simulink model "x35BusNetworkElectricityTransmissionModel"  (R2023b)
settings: Solver=VariableStepAuto  StartTime=0.0  StopTime=0.8  RelTol=1e-3
model workspace (MAT data in the model file):
  Compensation_Ki = 30
  Compensation_Kp = 3
  DC_Ki = 400
  DC_Kp = 8
  F = 0.01
  Flux_min = 0.5
  Grid_Freq_PWM = 2700
  Grid_Ireg_Ki = 5
  Grid_Ireg_Kp = 0.83
  Grid_Ireg_lim = 1.1
  Grid_Modindex_Upper = 1.1
  Grid_conv_Imax = 0.8
  H = 0.685
  Idref_max = 0.9
  Iqref_Tc = 0.3
  Ki_Var = 0.05
  Ki_Vreg = 20
  Ksh = 1.1
  L_pu = 0.3
  Llr = 0.16
  Lls = 0.18
  Lm = 2.9
  Nb_wt = 6
  P_mech = 1080000
  Pitch_Ki = 0
  Pitch_Kp = 150
  Pitch_Max = 27
  Pitch_Tc = 0.01
  Pitch_rate = 10
  Q_Filt = 50
  R_pu = 0.003
  Rotor_Freq_PWM = 1620
  Rotor_Ireg_Ki = 8
  Rotor_Ireg_Kp = 0.6
  Rotor_Ireg_lim = 0.1
  Rotor_Modindex_Upper = 2
  Rr = 0.016
  Rs = 0.023
  T_set = 0.0001
  Tp = 5e-05
  Ts = 5e-06
  Var_C_Filt = 720000
  Var_reg_max = 1.1
  Var_reg_min = 0.9
  WT_Coeff = [0.645 116 0.4 5 21 0.00912 0.08 0.035]
  WT_H = 4.32
  WT_IGBTRon = 5.931
  WT_Param = [91.204 10143]
  Wind_Freq_Filt = 10000
  Wind_Freq_nom = 60
  Wind_P_nom = 1200000
  Wind_Rotor_V_nom = 1950
  Wind_V_nom = 500
  Zeta_Filt = 0.707106781187
  init = [-0.2 0 0 0 0 0 0 0]
  p = 3
  torque0 = 0.83
  v_Ki = 0.1
  v_Kp = 3.6
  v_Max = 1.2
  v_Min = 0.7
  v_T = 5
  vreg_max = 1
  wind_VDC_nom = 1150
  wt0 = 1.2
undefined symbols (not defined in the file): D1, D11, Delta, DiscIntNeverNeededParam, Ion, Lithium, P, Q
libraries: powerlib_extras x144, spsSeriesRLCBranchLib x67, spsLoadFlowBusLib x43, spsThreePhaseTransformerTwoWindingsLib x32, spsThreePhaseSeriesRLCLoadLib x31, spsThreePhaseVIMeasurementLib x26, simulink_extras x26, spsDistributedParametersLineLib x22, spsGenericPowerSystemStabilizerLib x20, spsSynchronousMachinepuStandardLib x10, spsExcitationSystemLib x10, spsHydraulicTurbineandGovernorLib x10
(part 3 of 16)

== system x35BusNetworkElectricityTransmissionModel/North Network ==
  1320 MVar : spsThreePhaseSeriesRLCLoadLib/Three-Phase Series RLC Load  LConnTagsString=A|B|C  Configuration=Y (grounded)  NominalVoltage=650e3  Vabc=[1e3 1e3 1e3]  Vabcp=[1e3 1e3 1e3]  NominalFrequency=60  UnbalancedPower=off  ActivePower=4400e3  InductivePower=1320e6  CapacitivePower=0  Pabc=[10e3 9e3 11e3]  QLabc=[100 90 110]  QCabc=[100 90 110]  Pabcp=[10e3 9e3 11e3]  QLabcp=[100 90 110]  QCabcp=[100 90 110]  Measurements=None  LoadType=constant Z
  135 MW : spsThreePhaseSeriesRLCLoadLib/Three-Phase Series RLC Load  LConnTagsString=A|B|C  Configuration=Y (grounded)  NominalVoltage=17e3  Vabc=[1e3 1e3 1e3]  Vabcp=[1e3 1e3 1e3]  NominalFrequency=60  UnbalancedPower=off  ActivePower=135e6  InductivePower=0  CapacitivePower=0  Pabc=[10e3 9e3 11e3]  QLabc=[100 90 110]  QCabc=[100 90 110]  Pabcp=[10e3 9e3 11e3]  QLabcp=[100 90 110]  QCabcp=[100 90 110]  Measurements=None  LoadType=constant Z
  155 MW : spsThreePhaseSeriesRLCLoadLib/Three-Phase Series RLC Load  LConnTagsString=A|B|C  Configuration=Y (grounded)  NominalVoltage=17e3  Vabc=[1e3 1e3 1e3]  Vabcp=[1e3 1e3 1e3]  NominalFrequency=60  UnbalancedPower=off  ActivePower=155e6  InductivePower=0  CapacitivePower=0  Pabc=[10e3 9e3 11e3]  QLabc=[100 90 110]  QCabc=[100 90 110]  Pabcp=[10e3 9e3 11e3]  QLabcp=[100 90 110]  QCabcp=[100 90 110]  Measurements=None  LoadType=constant Z
  1980 MVar : spsThreePhaseSeriesRLCLoadLib/Three-Phase Series RLC Load  LConnTagsString=A|B|C  Configuration=Y (grounded)  NominalVoltage=650e3  Vabc=[1e3 1e3 1e3]  Vabcp=[1e3 1e3 1e3]  NominalFrequency=60  UnbalancedPower=off  ActivePower=6600e3  InductivePower=1980e6  CapacitivePower=0  Pabc=[10e3 9e3 11e3]  QLabc=[100 90 110]  QCabc=[100 90 110]  Pabcp=[10e3 9e3 11e3]  QLabcp=[100 90 110]  QCabcp=[100 90 110]  Measurements=None  LoadType=constant Z
  205 MW : spsThreePhaseSeriesRLCLoadLib/Three-Phase Series RLC Load  LConnTagsString=A|B|C  Configuration=Y (grounded)  NominalVoltage=17e3  Vabc=[1e3 1e3 1e3]  Vabcp=[1e3 1e3 1e3]  NominalFrequency=60  UnbalancedPower=off  ActivePower=205e6  InductivePower=0  CapacitivePower=0  Pabc=[10e3 9e3 11e3]  QLabc=[100 90 110]  QCabc=[100 90 110]  Pabcp=[10e3 9e3 11e3]  QLabcp=[100 90 110]  QCabcp=[100 90 110]  Measurements=None  LoadType=constant Z
  "2700 MVA 17KV :650KV Transformer " : spsThreePhaseTransformerTwoWindingsLib/Three-Phase Transformer (Two Windings)  Winding1Connection=Yg  Winding2Connection=Delta (D1)  CoreType=Three single-phase transformers  SetSaturation=off  Hysteresis=off  DataFile='hysteresis'  SetInitialFlux=off  Measurements=None  UNITS=pu  NominalPower=[ 2700e6 , 60 ]  Winding1=[650e3 , 0.002 , 0.08 ]  Winding2=[17e3 , 0.002 , 0.08 ]  Rm=500  Lm=500  L0=0.5  Saturation=[ 0,0 ; 0.0024,1.2 ; 1.0,1.52 ]  InitialFluxes=[ 0.8 , -0.8 , 0.7 ]  BreakLoop=off  DiscreteSolver=Trapezoidal iterative  DataType=off  TransfoNumber=1
  "3100 MVA 17KV :650KV Transformer " : spsThreePhaseTransformerTwoWindingsLib/Three-Phase Transformer (Two Windings)  Winding1Connection=Yg  Winding2Connection=Delta (D1)  CoreType=Three single-phase transformers  SetSaturation=off  Hysteresis=off  DataFile='hysteresis'  SetInitialFlux=off  Measurements=None  UNITS=pu  NominalPower=[ 3100e6 , 60 ]  Winding1=[ 650e3 , 0.002 , 0.08 ]  Winding2=[ 17e3 , 0.002 , 0.08 ]  Rm=500  Lm=500  L0=0.5  Saturation=[ 0,0 ; 0.0024,1.2 ; 1.0,1.52 ]  InitialFluxes=[ 0.8 , -0.8 , 0.7 ]  BreakLoop=off  DiscreteSolver=Trapezoidal iterative  DataType=off  TransfoNumber=1
  "4100 MVA 17KV :650KV Transformer " : spsThreePhaseTransformerTwoWindingsLib/Three-Phase Transformer (Two Windings)  Winding1Connection=Yg  Winding2Connection=Delta (D1)  CoreType=Three single-phase transformers  SetSaturation=off  Hysteresis=off  DataFile='hysteresis'  SetInitialFlux=off  Measurements=None  UNITS=pu  NominalPower=[ 4100e6 , 60 ]  Winding1=[ 650e3 , 0.002 , 0.08 ]  Winding2=[ 17e3 , 0.002 , 0.08 ]  Rm=500  Lm=500  L0=0.5  Saturation=[ 0,0 ; 0.0024,1.2 ; 1.0,1.52 ]  InitialFluxes=[ 0.8 , -0.8 , 0.7 ]  BreakLoop=off  DiscreteSolver=Trapezoidal iterative  DataType=off  TransfoNumber=1
  660 MVar : spsThreePhaseSeriesRLCLoadLib/Three-Phase Series RLC Load  LConnTagsString=A|B|C  Configuration=Y (grounded)  NominalVoltage=650e3  Vabc=[1e3 1e3 1e3]  Vabcp=[1e3 1e3 1e3]  NominalFrequency=60  UnbalancedPower=off  ActivePower=2200e3  InductivePower=660e6  CapacitivePower=0  Pabc=[10e3 9e3 11e3]  QLabc=[100 90 110]  QCabc=[100 90 110]  Pabcp=[10e3 9e3 11e3]  QLabcp=[100 90 110]  QCabcp=[100 90 110]  Measurements=None  LoadType=constant Z
  990 Mvar : spsThreePhaseParallelRLCLoadLib/Three-Phase Parallel RLC Load  LConnTagsString=A|B|C  Configuration=Y (grounded)  NominalVoltage=650e3  Vabc=[1e3 1e3 1e3]  Vabcp=[1e3 1e3 1e3]  NominalFrequency=60  UnbalancedPower=off  ActivePower=3300e3  InductivePower=990e6  CapacitivePower=0  Pabc=[10e3 9e3 11e3]  QLabc=[100 90 110]  QCabc=[100 90 110]  Pabcp=[10e3 9e3 11e3]  QLabcp=[100 90 110]  QCabcp=[100 90 110]  Measurements=None  LoadType=constant Z
  ATL-CAD 447 km : spsDistributedParametersLineLib/Distributed Parameters Line  Phases=3  Length=447  Frequency=60  Resistance=[0.01273 0.3864]/6  Inductance="[0.9337e-3  4.1264e-3]/6"  Capacitance=[12.74e-9 7.751e-9]*6  x1=[-0.00258 1.64377320763255e-08 -194904.094021767 -120223.665929989;-0.00252 1.80656414411054e-08 -192135.055279541 -124601.181939555;-0.00246 1.96843080899094e-08 -189267.716692787 -128914.949682076;-0.0024 2.12929038829704e-08 -186303.545244907 -133162.762154265;-0.00234 2.28906058329572e-08 -183244.057460786 -137342.44609677;-0.00228 2.44765965260301e-08 -180090.818630907 -141451.863106056;-0.00222 2.60500645400448e-08 -176845.442010521 -145488.910728447;-0.00216 2.7610204859691e-08 -173509.587994275 -149451.523535784;-0.0021 2.9156219288353e-08 -170084.963266721 -153337.674182133;-0.00204 3.06873168564822e-08 -166573.319929152 -157145.374441016;-0.00198 3.22027142262711e-08 -162976.454603186 -160872.676222622;-0.00192 3.37016360924241e-08 -159296.207511587 -164517.672570487;-0.00186 3.51833155788176e-08 -155534.461536769 -168078.498637129;-0.0018 3.6646994630848e-08 -151693.141257482 -171553.332638133;-0.00174 3.80919244032667e-08 -147774.211964161 -174940.39678422;-0.00168 3.95173656433029e-08 -143779.678653446 -178237.958190784;-0.00162 4.09225890688789e-08 -139711.585002389 -181444.329764479;-0.00156 4.23068757417249e-08 -135572.012322871 -184557.871066362;-0.0015 4.36695174352002e-08 -131363.078496766 -187576.989151169;-0.00144 4.50098169966357e-08 -127086.936892391 -190500.139382302;-0.00138 4.632708870401e-08 -122745.775262806 -193325.826222089;-0.00132 4.76206586167771e-08 -118341.814626515 -196052.603996931;-0.00126 4.88898649206673e-08 -113877.308131156 -198679.077636932;-0.0012 5.01340582662832e-08 -109354.539900746 -201203.903389647;-0.00114 5.13526021013192e-08 -104775.823867084 -203625.789507567;-0.00108 5.25448729962332e-08 -100143.502585896 -205943.496909003;-0.00102 5.37102609632047e-08 -95459.9460383467 -208155.839812022;-0.00096 5.48481697682159e-08 -90727.5504185068 -210261.686341115;-0.0009 5.5958017236096e-08 -85948.7369074205 -212259.959106288;-0.00084 5.70392355483729e-08 -81125.9504343822 -214149.635754268;-0.00078 5.80912715337793e-08 -76261.6584260665 -215929.749491566;-0.00072 5.91135869512658e-08 -71358.3495441466 -217599.389579101;-0.00066 6.01056587653745e-08 -66418.5324120493 -219157.701798153;-0.0006 6.1066979413834e-08 -61444.7343314965 -220603.888887397;-0.00054 6.19970570672373e-08 -56439.4999894916 -221937.210950794;-0.00048 6.28954158806711e-08 -51405.39015641 -223156.985836141;-0.00042 6.37615962371667e-08 -46344.980375862 -224262.589484067;-0.00036 6.45951549828486e-08 -41260.859646997 -225253.456247317;-0.0003 6.53956656536599e-08 -36155.6290999235 -226129.079180146;-0.00024 6.61627186935499e-08 -31031.9006649233 -226889.010297681;-0.00018 6.68959216640098e-08 -25892.2957361393 -227532.86080512;-0.00012 6.75948994448519e-08 -20739.4438304221 -228060.301296648;-6e-05 6.82592944261279e-08 -15575.9812420204 -228471.061923963]  x2=[-0.00258 4.87559476940855e-09 -301606.612191046 -117006.023986347;-0.00252 5.95262307883651e-09 -298883.042776193 -123797.71586053;-0.00246 7.02660591630551e-09 -296006.559273932 -130526.070535761;-0.0024 8.09699381235099e-09 -292978.633346374 -137187.64566146;-0.00234 9.16323913674683e-09 -289800.814136373 -143779.033052703;-0.00228 1.02247963786831e-08 -286474.727474956 -150296.860433905;-0.00222 1.12811224258595e-08 -283002.07504952 -156737.793164143;-0.00216 1.23316768423517e-08 -279384.63353321 -163098.535943216;-0.0021 1.33759221451082e-08 -275624.253675951 -169375.834497586;-0.00204 1.44133240789366e-08 -271722.85935756 -175566.477245322;-0.00198 1.54433518898386e-08 -267682.446603461 -181667.296939203;-0.00192 1.64654785965534e-08 -263505.082563477 -187675.172287145;-0.00186 1.74791812601711e-08 -259192.904454239 -193587.029549106;-0.0018 1.84839412516781e-08 -254748.118465748 -199399.844109673;-0.00174 1.94792445172967e-08 -250172.998632646 -205110.642025508;-0.00168 2.04645818414852e-08 -245469.885670778 -210716.501546873;-0.00162 2.14394491074616e-08 -240641.185779639 -216214.554612454;-0.00156 2.24033475551191e-08 -235689.369411317 -221601.98831671;-0.0015 2.33557840362012e-08 -230616.970006566 -226876.046349009;-0.00144 2.42962712666051e-08 -225426.582698647 -232034.030403808;-0.00138 2.52243280756855e-08 -220120.862985616 -237073.301561157;-0.00132 2.61394796524304e-08 -214702.525371715 -241991.281636816;-0.00126 2.70412577883831e-08 -209174.341978588 -246785.454501306;-0.0012 2.79292011171863e-08 -203539.141127007 -251453.367367201;-0.00114 2.88028553506256e-08 -197799.805889854 -255992.632044027;-0.00108 2.96617735110519e-08 -191959.272617088 -260400.9261601;-0.00102 3.05055161600635e-08 -186020.529433451 -264675.994350693;-0.00096 3.13336516233304e-08 -179986.614709693 -268815.649411926;-0.0009 3.21457562114475e-08 -173860.615508078 -272817.773419778;-0.00084 3.29414144367015e-08 -167645.666002995 -276680.318813656;-0.00078 3.37202192256424e-08 -161344.945877449 -280401.309443964;-0.00072 3.44817721273494e-08 -154961.67869628 -283978.84158314;-0.00066 3.52256835172862e-08 -148499.130256927 -287411.084899637;-0.0006 3.59515727966398e-08 -141960.606918587 -290696.283394352;-0.00054 3.66590685870419e-08 -135349.453910617 -293832.756299034;-0.00048 3.73478089205732e-08 -128669.053621055 -296818.898936187;-0.00042 3.80174414249525e-08 -121922.823866131 -299653.183540063;-0.00036 3.86676235038173e-08 -115114.216141641 -302334.160038285;-0.0003 3.9298022512002e-08 -108246.713857108 -304860.456793738;-0.00024 3.99083159257256e-08 -101323.830553596 -307230.781306322;-0.00018 4.04981915076007e-08 -94349.1081061232 -309443.920874218;-0.00012 4.106734746638e-08 -87326.1149115726 -311498.743214328;-6e-05 4.16154926113581e-08 -80258.4440630321 -313394.197041575]  x3=[-0.00258 2.91635300112185e-11 -5053.27339398635 2918.21649596622;-0.00252 3.84630024253407e-11 -5117.98290026042 2803.17747700594;-0.00246 4.77427964567074e-11 -5180.07395191326 2686.70430065166;-0.0024 5.69981643912216e-11 -5239.51478201554 2568.85655673258;-0.00234 6.62243710116282e-11 -5296.27497954025 2449.69453833206;-0.00228 7.54166960201396e-11 -5350.3255049215 2329.27921094058;-0.00222 8.45704364534267e-11 -5401.6387049118 2207.67218126465;-0.00216 9.36809090887422e-11 -5450.18832672985 2084.9356657077;-0.0021 1.02743452839944e-10 -5495.94953149205 1961.13245853899;-0.00204 1.11753431142192e-10 -5538.89890692046 1836.32589976693;-0.00198 1.20706234324102e-10 -5579.01447932101 1710.57984273314;-0.00192 1.29597281966136e-10 -5616.2757248256 1583.95862144394;-0.00186 1.38422025244034e-10 -5650.66357989254 1456.52701765581;-0.0018 1.47175949256073e-10 -5682.16045105973 1328.35022773192;-0.00174 1.55854575332973e-10 -5710.75022394592 1199.49382928644;-0.00168 1.64453463329272e-10 -5736.418271495 1070.0237476338;-0.00162 1.7296821389498e-10 -5759.15146145956 940.006222060097;-0.00156 1.81394470726375e-10 -5778.93816311956 809.507771933874;-0.0015 1.89727922794762e-10 -5795.7682532328 678.595162673546;-0.00144 1.97964306552078e-10 -5809.63312121421 547.335371588997;-0.00138 2.06099408112202e-10 -5820.52567354113 415.795553614749;-0.00132 2.14129065406857e-10 -5828.44033738251 284.043006952253;-0.00126 2.22049170315e-10 -5833.37306345009 152.145138638889;-0.0012 2.29855670764612e-10 -5835.32132807008 20.1694300612777;-0.00114 2.37544572805817e-10 -5834.28413447428 -111.816597569441;-0.00108 2.45111942654255e-10 -5830.26201331011 -243.745417762709;-0.00102 2.52553908703683e-10 -5823.25702236907 -375.549533296353;-0.00096 2.59866663506759e-10 -5813.27274553397 -507.161510749404;-0.0009 2.67046465723001e-10 -5800.31429094533 -638.51401500229;-0.00084 2.74089642032928e-10 -5784.38828838795 -769.539843686717;-0.00078 2.80992589017397e-10 -5765.50288589903 -900.171961567653;-0.00072 2.87751775001178e-10 -5743.66774559943 -1030.34353483979;-0.00066 2.94363741859827e-10 -5718.89403875042 -1159.98796532093;-0.0006 3.00825106788924e-10 -5691.19444003816 -1289.03892452491;-0.00054 3.07132564034779e-10 -5660.5831210892 -1417.4303875964;-0.00048 3.13282886585716e-10 -5627.07574321994 -1545.0966670905;-0.00042 3.19272927823074e-10 -5590.68944942404 -1671.9724465796;-0.00036 3.25099623131072e-10 -5551.44285560176 -1797.99281407054;-0.0003 3.30759991464727e-10 -5509.35604103568 -1923.09329521471;-0.00024 3.36251136875005e-10 -5464.45053811781 -2047.20988629437;-0.00018 3.41570249990452e-10 -5416.7493213332 -2170.27908696812;-0.00012 3.46714609454512e-10 -5366.27679550578 -2292.23793275882;-6e-05 3.51681583317825e-10 -5313.05878331239 -2413.02402726744]  x4=[-0.00258 -3.35866188879571e-10 -7329.89893613951 -4834.75933302617;-0.00252 -3.24943372678954e-10 -7218.67296251981 -4999.30757604478;-0.00246 -3.13854309444611e-10 -7103.75378242676 -5161.29808093091;-0.0024 -3.02604672546196e-10 -6985.20019063633 -5320.647970349;-0.00234 -2.91200217505814e-10 -6863.07284135671 -5477.2757179512;-0.00228 -2.79646779053395e-10 -6737.43421719646 -5631.10119008767;-0.00222 -2.67950268141535e-10 -6608.34859719721 -5782.04568680451;-0.00216 -2.56116668921341e-10 -6475.8820239474 -5930.03198210806;-0.0021 -2.44152035680835e-10 -6340.10226979359 -6074.98436347517;-0.00204 -2.32062489747464e-10 -6201.07880216694 -6216.82867058912;-0.00198 -2.19854216356316e-10 -6058.88274804233 -6355.49233328141;-0.00192 -2.07533461485642e-10 -5913.58685754855 -6490.90440866;-0.00186 -1.95106528661294e-10 -5765.26546674792 -6622.99561740499;-0.0018 -1.82579775731729e-10 -5613.99445960465 -6751.69837921324;-0.00174 -1.69959611615213e-10 -5459.85122916116 -6876.94684737363;-0.00168 -1.57252493020902e-10 -5302.91463794237 -6998.67694245554;-0.00162 -1.4446492114547e-10 -5143.26497760822 -7116.82638509301;-0.00156 -1.31603438346975e-10 -4980.98392787491 -7231.33472784804;-0.0015 -1.1867462479767e-10 -4816.1545147261 -7342.14338613659;-0.00144 -1.05685095117463e-10 -4648.86106793525 -7449.19566820159;-0.00138 -9.26414949897582e-11 -4479.18917792097 -7552.43680411743;-0.00132 -7.95504977613986e-11 -4307.22565195737 -7651.81397381129;-0.00126 -6.641880102846e-11 -4133.05846976185 -7747.27633408688;-0.0012 -5.3253123209637e-11 -3956.77673848305 -7838.77504463675;-0.00114 -4.00602001089753e-11 -3778.47064711202 -7926.26329302987;-0.00108 -2.68467814697105e-11 -3598.23142033982 -8009.69631866178;-0.00102 -1.36196275209744e-11 -3416.1512718853 -8089.03143565488;-0.00096 -3.85505519136652e-13 -3232.32335731687 -8164.22805469739;-0.0009 1.2848813714448e-11 -3046.84172639237 -8235.24770380952;-0.00084 2.60765592575175e-11 -2859.80127494148 -8302.05404802651;-0.00078 3.92909635510314e-11 -2671.29769631527 -8364.6129079882;-0.00072 5.24852658615791e-11 -2481.42743242773 -8422.89227742589;-0.00066 6.56527157402959e-11 -2290.28762441425 -8476.8623395373;-0.0006 7.87865764765172e-11 -2097.97606293247 -8526.49548224139;-0.00054 9.18801285444045e-11 -1904.59113813076 -8571.76631230524;-0.00048 1.04926673040779e-10 -1710.23178930997 -8612.65166833569;-0.00042 1.17919535112404e-10 -1514.99745430433 -8649.13063262912;-0.00036 1.30852067370963e-10 -1318.98801860713 -8681.18454187333;-0.0003 1.43717653293986e-10 -1122.30376426752 -8708.79699669608;-0.00024 1.56509710609988e-10 -925.045318584315 -8731.95387005524;-0.00018 1.69221694666074e-10 -727.313602623252 -8750.64331446653;-0.00012 1.81847101776312e-10 -529.209779583876 -8764.85576806484;-6e-05 1.94379472549133e-10 -330.835203042593 -8774.5839594963]  x5=0.00252797080447097  V1=[6.404e-19 2.341e-08 2.341e-08;377 377 377;-1.588 0.8733 -0.6975]  V2=[3.447e-16 8.016e-05 8.016e-05;377 377 377;2.581 0.8892 -0.6816]  I1=[4.995e-19 5.332e-07 5.332e-07;377 377 377;1.203 -0.6479 -2.219]  I2=[4.022e-19 5.225e-07 5.225e-07;377 377 377;-2.95 1.909 0.3385]  nHarmo=1  Measurements=None  Decoupling=off  VsMag0=0  VrMag0=0  VsAngle0=0  VrAngle0=0  IsMag0=0  IrMag0=0  IsAngle0=0  IrAngle0=0
      settings: LibrarySourceBlock=sps_lib/Power Grid Elements/Distributed Parameters Line
  BMW 1 : spsThreePhaseVIMeasurementLib/Three-Phase V-I Measurement  VoltageMeasurement=no  SetLabelV=off  LabelV=Vabc  Vpu=off  VpuLL=off  CurrentMeasurement=no  SetLabelI=off  LabelI=Iabc  Ipu=off  Pbase=100e6  Vbase=500e3  OutputType=Complex  PhasorSimulation=off  PSBequivalent=0
  BMW- FER 131 km : spsDistributedParametersLineLib/Distributed Parameters Line  Phases=3  Length=131  Frequency=60  Resistance=[0.01273 0.3864]/6  Inductance="[0.9337e-3  4.1264e-3]/6"  Capacitance=[12.74e-9 7.751e-9]*6  x1=[-0.00078 5.80912715337793e-08 -76261.6584260665 -215929.749491566;-0.00072 5.91135869512658e-08 -71358.3495441466 -217599.389579101;-0.00066 6.01056587653745e-08 -66418.5324120492 -219157.701798153;-0.0006 6.1066979413834e-08 -61444.7343314965 -220603.888887397;-0.00054 6.19970570672373e-08 -56439.4999894916 -221937.210950794;-0.00048 6.28954158806711e-08 -51405.39015641 -223156.985836141;-0.00042 6.37615962371667e-08 -46344.980375862 -224262.589484067;-0.00036 6.45951549828486e-08 -41260.859646997 -225253.456247317;-0.0003 6.53956656536599e-08 -36155.6290999235 -226129.079180146;-0.00024 6.61627186935499e-08 -31031.9006649233 -226889.010297681;-0.00018 6.68959216640098e-08 -25892.2957361393 -227532.86080512;-0.00012 6.75948994448519e-08 -20739.4438304221 -228060.301296648;-6e-05 6.82592944261279e-08 -15575.9812420204 -228471.061923963]  x2=[-0.00078 2.91154256756996e-08 -40332.3471165906 -195014.245406608;-0.00072 3.00931854241187e-08 -35911.2883875951 -195876.599881198;-0.00066 3.10555489428166e-08 -31471.8567798962 -196638.740267906;-0.0006 3.20020238688349e-08 -27016.3235887357 -197300.276641627;-0.00054 3.29321259681124e-08 -22546.9683472229 -197860.870548128;-0.00048 3.3845379383229e-08 -18066.0776600836 -198320.235177208;-0.00042 3.47413168768623e-08 -13575.9440337906 -198678.135509435;-0.00036 3.56194800708358e-08 -9078.86470367538 -198934.388436385;-0.0003 3.64794196806327e-08 -4577.1404586196 -199088.862854326;-0.00024 3.73206957452588e-08 -73.0744639293679 -199141.479731292;-0.00018 3.81428778523344e-08 4431.02891700687 -199092.212147516;-0.00012 3.89455453583015e-08 8932.86530167318 -198941.085309204;-6e-05 3.97282876036323e-08 13430.1314673908 -198688.17653564]  x3=[-0.00078 2.7051916331608e-10 801.205877154994 -9199.13249771914;-0.00072 2.61865618398496e-10 1009.06227174107 -9178.65876986299;-0.00066 2.53078098191819e-10 1216.40241142359 -9153.48907057806;-0.0006 2.44161098553761e-10 1423.1202171559 -9123.63627714759;-0.00054 2.35119181586105e-10 1629.10992828887 -9089.11566281232;-0.00048 2.25956973300646e-10 1834.26615668004 -9049.9448889564;-0.00042 2.16679161252442e-10 2038.48394061211 -9006.14399607155;-0.00036 2.07290492141571e-10 2241.65879849331 -8957.73539350389;-0.0003 1.97795769384632e-10 2443.68678231211 -8904.743847989;-0.00024 1.8819985065723e-10 2644.46453081894 -8847.19647098073;-0.00018 1.78507645408699e-10 2843.88932240772 -8785.12270478051;-0.00012 1.68724112350334e-10 3041.85912767011 -8718.55430747412;-6e-05 1.58854256918428e-10 3238.2726615957 -8647.52533668367]  x4=[-0.00078 3.05744357291441e-10 -4148.52157769771 353.308180522301;-0.00072 3.32262569637252e-10 -4155.45083096756 259.388186850742;-0.00066 3.5861079031293e-10 -4160.25407880839 165.335485389847;-0.0006 3.84775539081918e-10 -4162.92886378985 71.1981952395781;-0.00054 4.10743429575277e-10 -4163.4738174425 -22.9755212229666;-0.00048 4.365011761404e-10 -4161.888660958 -117.137482984315;-0.00042 4.62035600638195e-10 -4158.1742053317 -211.239515044916;-0.00036 4.87333639185267e-10 -4152.33235094772 -305.233473066364;-0.0003 5.12382348837641e-10 -4144.36608660672 -399.071268002924;-0.00024 5.37168914212613e-10 -4134.27948799673 -492.704890704785;-0.00018 5.61680654045334e-10 -4122.07771560798 -586.086436480422;-0.00012 5.8590502767678e-10 -4107.76701209269 -679.168129605523;-6e-05 6.09829641469786e-10 -4091.3546990712 -771.902347765934]  x5=0.000740859452764423  V1=[1.271e-18 2.341e-08 2.341e-08;377 377 377;2.226 1.284 -0.2866]  V2=[3.351e-20 3.07e-09 3.07e-09;377 377 377;-0.6702 -1.817 2.896]  I1=[5.66e-21 5.705e-10 5.705e-10;377 377 377;-2.518 2.745 1.174]  I2=[6.071e-21 5.74e-10 5.74e-10;377 377 377;0.8934 -0.2657 -1.836]  nHarmo=1  Measurements=None  Decoupling=off  VsMag0=0  VrMag0=0  VsAngle0=0  VrAngle0=0  IsMag0=0  IrMag0=0  IsAngle0=0  IrAngle0=0
      settings: LibrarySourceBlock=sps_lib/Power Grid Elements/Distributed Parameters Line
  BMW- ORE 215 km : spsDistributedParametersLineLib/Distributed Parameters Line  Phases=3  Length=215  Frequency=60  Resistance=[0.01273 0.3864]/6  Inductance="[0.9337e-3  4.1264e-3]/6"  Capacitance=[12.74e-9 7.751e-9]*6  x1=[-0.00126 4.88898649206673e-08 -113877.308131156 -198679.077636932;-0.0012 5.01340582662832e-08 -109354.539900746 -201203.903389647;-0.00114 5.13526021013192e-08 -104775.823867084 -203625.789507567;-0.00108 5.25448729962332e-08 -100143.502585896 -205943.496909003;-0.00102 5.37102609632047e-08 -95459.9460383467 -208155.839812022;-0.00096 5.48481697682159e-08 -90727.5504185068 -210261.686341115;-0.0009 5.5958017236096e-08 -85948.7369074205 -212259.959106288;-0.00084 5.70392355483729e-08 -81125.9504343822 -214149.635754268;-0.00078 5.80912715337793e-08 -76261.6584260665 -215929.749491566;-0.00072 5.91135869512658e-08 -71358.3495441466 -217599.389579101;-0.00066 6.01056587653745e-08 -66418.5324120492 -219157.701798153;-0.0006 6.1066979413834e-08 -61444.7343314965 -220603.888887397;-0.00054 6.19970570672373e-08 -56439.4999894916 -221937.210950794;-0.00048 6.28954158806711e-08 -51405.39015641 -223156.985836141;-0.00042 6.37615962371667e-08 -46344.980375862 -224262.589484067;-0.00036 6.45951549828486e-08 -41260.859646997 -225253.456247317;-0.0003 6.53956656536599e-08 -36155.6290999235 -226129.079180146;-0.00024 6.61627186935499e-08 -31031.9006649233 -226889.010297681;-0.00018 6.68959216640098e-08 -25892.2957361393 -227532.86080512;-0.00012 6.75948994448519e-08 -20739.4438304221 -228060.301296648;-6e-05 6.82592944261279e-08 -15575.9812420204 -228471.061923963]  x2=[-0.00126 1.36103658168936e-08 -202813.109882575 -207023.441617023;-0.0012 1.38562428628494e-08 -198078.85681003 -211557.646069082;-0.00114 1.40950307989227e-08 -193243.262934264 -215983.613720276;-0.00108 1.4326607456793e-08 -188308.802234456 -220299.080163773;-0.00102 1.45508543575631e-08 -183277.999271879 -224501.837527199;-0.00096 1.4767656772375e-08 -178153.427898286 -228589.735602229;-0.0009 1.49769037811073e-08 -172937.709939083 -232560.682944673;-0.00084 1.51784883291238e-08 -167633.513851954 -236412.647944494;-0.00078 1.53723072820449e-08 -162243.553361628 -240143.659865224;-0.00072 1.55582614785129e-08 -156770.586071485 -243751.809852222;-0.00066 1.57362557809248e-08 -151217.412052721 -247235.251909284;-0.0006 1.59061991241067e-08 -145586.872411774 -250592.203843087;-0.00054 1.6068004561904e-08 -139881.847836765 -253820.948174992;-0.00048 1.62215893116647e-08 -134105.257123683 -256919.833019739;-0.00042 1.63668747965932e-08 -128260.055683077 -259887.272930581;-0.00036 1.65037866859506e-08 -122349.23402801 -262721.749710426;-0.0003 1.66322549330845e-08 -116375.81624406 -265421.81318858;-0.00024 1.6752213811266e-08 -110342.858442142 -267986.081962676;-0.00018 1.68636019473163e-08 -104253.447194943 -270413.244105426;-0.00012 1.69663623530068e-08 -98110.6979577777 -272702.057835829;-6e-05 1.70604424542152e-08 -91917.7534746594 -274851.352154489]  x3=[-0.00126 8.69836358039925e-10 -4039.64980114856 3058.27670176948;-0.0012 8.63889633892926e-10 -4107.7865446866 2966.12730134233;-0.00114 8.57500927846383e-10 -4173.82166872521 2872.46037538009;-0.00108 8.50673508480359e-10 -4237.72138847475 2777.32384561284;-0.00102 8.43410868828756e-10 -4299.45301165785 2680.76638564712;-0.00096 8.3571672459222e-10 -4358.98495523544 2582.83739606364;-0.0009 8.27595012237113e-10 -4416.28676156514 2483.58697914299;-0.00084 8.19049886981548e-10 -4471.32911398403 2383.0659132324;-0.00078 8.10085720669502e-10 -4524.08385180755 2281.3256267666;-0.00072 8.00707099534097e-10 -4574.52398473702 2178.4181719561;-0.00066 7.90918821851205e-10 -4622.62370666841 2074.39619815628;-0.0006 7.80725895484555e-10 -4668.35840889521 1969.31292493106;-0.00054 7.70133535323619e-10 -4711.70469269867 1863.22211482472;-0.00048 7.59147160615579e-10 -4752.64038131906 1756.17804585605;-0.00042 7.47772392192742e-10 -4791.14453130166 1648.23548374868;-0.00036 7.36015049596814e-10 -4827.19744321188 1539.44965391193;-0.0003 7.23881148101518e-10 -4860.7806717138 1429.87621318649;-0.00024 7.11376895635068e-10 -4891.87703500717 1319.5712213693;-0.00018 6.98508689604076e-10 -4920.47062361794 1208.59111253239;-0.00012 6.85283113620527e-10 -4946.54680853782 1096.99266615011;-6e-05 6.71706934133474e-10 -4970.09224870877 984.832978049736]  x4=[-0.00126 -5.19223589158569e-10 -4184.55199868995 -10999.0722268337;-0.0012 -4.99570046723291e-10 -3934.70964350595 -11090.9038546552;-0.00114 -4.79660915021117e-10 -3682.85421816326 -11177.0611711283;-0.00108 -4.59506379931703e-10 -3429.11457655123 -11257.5000965779;-0.00102 -4.39116752887615e-10 -3173.62053655909 -11332.1794769634;-0.00096 -4.18502465598804e-10 -2916.50281365868 -11401.0611049339;-0.0009 -3.97674064715557e-10 -2657.89295402802 -11464.1097393757;-0.00084 -3.7664220643263e-10 -2397.92326724987 -11521.2931234424;-0.00078 -3.55417651037343e-10 -2136.72675861967 -11572.5820010582;-0.00072 -3.34011257404423e-10 -1874.43706109759 -11617.9501318855;-0.00066 -3.12433977440396e-10 -1611.18836693943 -11657.3743047503;-0.0006 -2.90696850480395e-10 -1347.11535904141 -11690.8343495173;-0.00054 -2.68810997640228e-10 -1082.35314203388 -11718.3131474093;-0.00048 -2.46787616126612e-10 -817.037173159289 -11739.7966397656;-0.00042 -2.24637973508475e-10 -551.303192969803 -11755.2738352344;-0.00036 -2.02373401952258e-10 -285.287155879882 -11764.7368153967;-0.0003 -1.80005292424172e-10 -19.1251606095117 -11768.1807388168;-0.00024 -1.57545088862366e-10 247.046619446418 -11765.60384352;-0.00018 -1.35004282322e-10 513.092005886943 -11757.0074478935;-0.00012 -1.12394405096206e-10 778.874884976406 -11742.3959500121;-6e-05 -8.97270248159542e-11 1044.25927728276 -11721.7768253882]  x5=0.00121591436904085  V1=[1.271e-18 2.341e-08 2.341e-08;377 377 377;2.047 1.175 -0.3959]  V2=[2.813e-15 0.004697 0.004697;377 377 377;-0.9882 1.143 -0.4279]  I1=[7.991e-18 6.252e-05 6.252e-05;377 377 377;-2.327 -0.3924 -1.963]  I2=[7.132e-18 6.19e-05 6.19e-05;377 377 377;0.3426 2.469 0.8982]  nHarmo=1  Measurements=None  Decoupling=off  VsMag0=0  VrMag0=0  VsAngle0=0  VrAngle0=0  IsMag0=0  IrMag0=0  IsAngle0=0  IrAngle0=0
      settings: LibrarySourceBlock=sps_lib/Power Grid Elements/Distributed Parameters Line
  CAD 3 : spsThreePhaseVIMeasurementLib/Three-Phase V-I Measurement  VoltageMeasurement=no  SetLabelV=off  LabelV=Vabc  Vpu=off  VpuLL=off  CurrentMeasurement=no  SetLabelI=off  LabelI=Iabc  Ipu=off  Pbase=100e6  Vbase=500e3  OutputType=Complex  PhasorSimulation=off  PSBequivalent=0
  Cs BMW- MPP8 : Subsystem
  Cs BMWN : Subsystem
  Cs FER : Subsystem
  Cs LTNN : Subsystem
  Cs ORED : Subsystem
  FER-LTN 78 km : spsDistributedParametersLineLib/Distributed Parameters Line  Phases=3  Length=78  Frequency=60  Resistance=[0.01273 0.3864]/6  Inductance="[0.9337e-3  4.1264e-3]/6"  Capacitance=[12.74e-9 7.751e-9]*6  x1=[-0.00048 3.870410165105e-08 0 0;-0.00042 3.95723935786357e-08 0 0;-0.00036 4.04204395384528e-08 0 0;-0.0003 4.12478056545182e-08 -25938.8871287904 -220720.061917529;-0.00024 4.2054068631039e-08 -20940.1114048065 -221250.298288259;-0.00018 4.28388159689782e-08 -15930.6223328991 -221667.338918148;-0.00012 4.36016461770974e-08 -10912.9828602421 -221970.970441506;-6e-05 4.43421689773666e-08 -5889.76010390505 -222161.037514834]  x2=[-0.00048 2.14936519483332e-08 0 0;-0.00042 2.2377103916222e-08 0 0;-0.00036 2.32491073442659e-08 0 0;-0.0003 2.41092160993983e-08 -7154.19773139822 -204077.139448111;-0.00024 2.49569901340873e-08 -2536.64996729834 -204186.767536818;-0.00018 2.57919957114715e-08 2082.19559379672 -204191.929902316;-0.00012 2.66138056272683e-08 6699.97586515144 -204092.623903444;-6e-05 2.74219994283398e-08 11314.3283050522 -203888.900346983]  x3=[-0.00048 5.98567264033076e-11 0 0;-0.00042 4.97546802891367e-11 0 0;-0.00036 3.96271787611692e-11 0 0;-0.0003 2.94794032363213e-11 2958.67727109397 -8817.493143416;-0.00024 1.9316545504061e-11 3157.34983991285 -8748.32024470552;-0.00018 9.14380507019212e-12 3354.40705021252 -8674.67154370749;-0.00012 -1.03361350330879e-12 3549.74808388299 -8596.58472045819;-6e-05 -1.12105032610424e-11 3743.27300084194 -8514.09972561928]  x4=[-0.00048 3.66938090062692e-10 0 0;-0.00042 3.91991483703486e-10 0 0;-0.00036 4.16844327258047e-10 0 0;-0.0003 4.41483905552385e-10 -4167.06026595294 -534.328418344685;-0.00024 4.65897612522958e-10 -4153.90868260721 -628.440741000594;-0.00018 4.90072957666166e-10 -4138.63188282404 -722.231541761157;-0.00012 5.13997572428726e-10 -4121.2376824965 -815.652835519651;-6e-05 5.37659216535647e-10 -4101.73498081888 -908.656826215961]  x5=0.000441122422256679  V1=[6.391e-24 5.815e-13 5.815e-13;377 377 377;2.579 1.39 -0.1804]  V2=[2.845e-25 1.398e-13 1.398e-13;377 377 377;-0.3188 -1.706 3.006]  I1=[5.031e-26 2.613e-14 2.613e-14;377 377 377;-2.041 2.924 1.353]  I2=[5.244e-26 2.622e-14 2.622e-14;377 377 377;1.254 -0.1553 -1.726]  nHarmo=1  Measurements=None  Decoupling=off  VsMag0=0  VrMag0=0  VsAngle0=0  VrAngle0=0  IsMag0=0  IrMag0=0  IsAngle0=0  IrAngle0=0
      settings: LibrarySourceBlock=sps_lib/Power Grid Elements/Distributed Parameters Line
  LTN 3 : spsThreePhaseVIMeasurementLib/Three-Phase V-I Measurement  VoltageMeasurement=no  SetLabelV=off  LabelV=Vabc  Vpu=off  VpuLL=off  CurrentMeasurement=no  SetLabelI=off  LabelI=Iabc  Ipu=off  Pbase=100e6  Vbase=500e3  OutputType=Complex  PhasorSimulation=off  PSBequivalent=0
  Load Flow Bus : spsLoadFlowBusLib/Load Flow Bus  LConnTagsString=a  Phases=single  Connectors=on one side  ID=BUS_13  Vbase=17e3  Vref=1  Vangle=0  VLF=1  VLFb=1  VLFc=1  angleLF=0  angleLFb=0  angleLFc=0
  Load Flow Bus1 : spsLoadFlowBusLib/Load Flow Bus  LConnTagsString=a  Phases=single  Connectors=on one side  ID=BUS_14  Vbase=650e3  Vref=1  Vangle=0  VLF=1  VLFb=1  VLFc=1  angleLF=0  angleLFb=0  angleLFc=0
  Load Flow Bus2 : spsLoadFlowBusLib/Load Flow Bus  LConnTagsString=a  Phases=single  Connectors=on one side  ID=BUS_15  Vbase=17e3  Vref=1  Vangle=0  VLF=1  VLFb=1  VLFc=1  angleLF=0  angleLFb=0  angleLFc=0
  Load Flow Bus3 : spsLoadFlowBusLib/Load Flow Bus  LConnTagsString=a  Phases=single  Connectors=on one side  ID=BUS_16  Vbase=650e3  Vref=1  Vangle=0  VLF=1  VLFb=1  VLFc=1  angleLF=0  angleLFb=0  angleLFc=0
  Load Flow Bus4 : spsLoadFlowBusLib/Load Flow Bus  LConnTagsString=a  Phases=single  Connectors=on one side  ID=BUS_17  Vbase=17e3  Vref=1  Vangle=0  VLF=1  VLFb=1  VLFc=1  angleLF=0  angleLFb=0  angleLFc=0
  Load Flow Bus6 : spsLoadFlowBusLib/Load Flow Bus  LConnTagsString=a  Phases=single  Connectors=on one side  ID=BUS_18  Vbase=650e3  Vref=1  Vangle=0  VLF=1  VLFb=1  VLFc=1  angleLF=0  angleLFb=0  angleLFc=0
  Load Flow Bus7 : spsLoadFlowBusLib/Load Flow Bus  LConnTagsString=a  Phases=single  Connectors=on one side  ID=BUS_19  Vbase=650e3  Vref=1  Vangle=0  VLF=1  VLFb=1  VLFc=1  angleLF=0  angleLFb=0  angleLFc=0
  Load Flow Bus8 : spsLoadFlowBusLib/Load Flow Bus  LConnTagsString=a  Phases=single  Connectors=on one side  ID=BUS_20  Vbase=650e3  Vref=1  Vangle=0  VLF=1  VLFb=1  VLFc=1  angleLF=0  angleLFb=0  angleLFc=0
  MPP7 2700 MVA 17KV : spsSynchronousMachinepuStandardLib/Synchronous Machine pu Standard  PresetModel=No  MechanicalLoad=Mechanical power Pm  ShowDetailedParameters=on  RotorType=Salient-pole  Units=per unit standard parameters  MeasurementBus=off  NominalParameters=[2700e6 17000 60]  Reactances1=[ 1.81, 0.3, 0.23, 1.76, 0.65, 0.25, 0.15 ]  Reactances2=[ 1.305, 0.296, 0.252, 0.474, 0.243, 0.18 ]  dAxisTimeConstants=Short-circuit  qAxisTimeConstants=Open-circuit  TimeConstants1="[ 4.4849  0.0681  0.1  ]"  TimeConstants2=[ 8.0, 0.03, 1.0, 0.07 ]  TimeConstants3="[  4.49  0.0681  0.0513  ]"  TimeConstants4=[ 8.0, 0.03, 0.3371, 0.0295 ]  TimeConstants5=[ 1.01, 0.053, 0.1 ]  TimeConstants6=[ 1.3201, 0.023, 1.0, 0.07 ]  TimeConstants7=[0.012 0.003 0.003]  TimeConstants8=[ 1.3201, 0.0231, 0.3371, 0.0295 ]  StatorResistance=2.8544e-3  Mechanical=[3.5 0 32]  PolePairs=20  InitialConditions=[0 -81.9543 0.907703 0.907703 0.907703 -8.76021 -128.76 111.24 1.25655]  SetSaturation=off  Saturation=[0.6404,0.7127,0.8441,0.9214,0.9956,1.082,1.19,1.316,1.457;0.7,0.7698,0.8872,0.9466,0.9969,1.046,1.1,1.151,1.201]  LoadFlowParameters=[1,0,0,0,0]  TsPowergui=0  TsBlock=-1  IterativeModel=Trapezoidal non iterative  IterativeDiscreteModel=Trapezoidal non iterative  BusType=PV  Pref=2200e6  Qref=0  Qmin=-inf  Qmax=inf  PLF=0  QLF=0
  MPP7-BMW 330 km : spsDistributedParametersLineLib/Distributed Parameters Line  Phases=3  Length=330  Frequency=60  Resistance=[0.01273 0.3864]/6  Inductance="[0.9337e-3  4.1264e-3]/6"  Capacitance=[12.74e-9 7.751e-9]*6  x1=[-0.00192 1.19950768751019e-07 0 0;-0.00186 1.22929423385072e-07 0 0;-0.0018 1.25845185054646e-07 0 0;-0.00174 1.28696562002195e-07 0 0;-0.00168 1.31482095410585e-07 0 0;-0.00162 1.34200360149452e-07 0 0;-0.00156 1.3684996550433e-07 0 0;-0.0015 1.39429555888159e-07 0 0;-0.00144 1.41937811534833e-07 0 0;-0.00138 1.44373449174417e-07 0 0;-0.00132 1.46735222689689e-07 0 0;-0.00126 1.49021923753678e-07 0 0;-0.0012 1.51232382447866e-07 0 0;-0.00114 1.5336546786074e-07 -132088.660854457 -207604.180723548;-0.00108 1.55420088666389e-07 -127359.369588715 -210538.620970177;-0.00102 1.57395193682843e-07 -122564.91891616 -213365.345768011;-0.00096 1.5928977240988e-07 -117707.761766349 -216082.908912412;-0.0009 1.61102855546015e-07 -112790.383150628 -218689.920047861;-0.00084 1.62833515484415e-07 -107815.298890761 -221185.045379288;-0.00078 1.64480866787476e-07 -102785.054331784 -223567.008354469;-0.00072 1.66044066639831e-07 -97702.2230397616 -225834.590317133;-0.00066 1.67522315279551e-07 -92569.4054851023 -227986.631130447;-0.0006 1.68914856407318e-07 -87389.2277121108 -230022.029770566;-0.00054 1.70220977573359e-07 -82164.3399954546 -231939.744889936;-0.00048 1.71440010541952e-07 -76897.4154842342 -233738.795350066;-0.00042 1.72571331633305e-07 -71591.1488343513 -235418.2607235;-0.00036 1.73614362042642e-07 -66248.2548298723 -236977.281764717;-0.0003 1.74568568136333e-07 -60871.4669940954 -238415.060849748;-0.00024 1.7543346172491e-07 -55463.536191029 -239730.862384243;-0.00018 1.76208600312831e-07 -50027.2292179988 -240924.013179826;-0.00012 1.76893587324871e-07 -44565.3273901039 -241993.902798502;-6e-05 1.77488072309018e-07 -39080.6251172436 -242939.983864973]  x2=[-0.00192 1.12654364208366e-07 0 0;-0.00186 1.14140058242287e-07 0 0;-0.0018 1.15567356113346e-07 0 0;-0.00174 1.16935527589578e-07 0 0;-0.00168 1.18243872689175e-07 0 0;-0.00162 1.19491722038609e-07 0 0;-0.00156 1.20678437215094e-07 0 0;-0.0015 1.2180341107322e-07 0 0;-0.00144 1.22866068055572e-07 0 0;-0.00138 1.23865864487202e-07 0 0;-0.00132 1.24802288853784e-07 0 0;-0.00126 1.25674862063306e-07 0 0;-0.0012 1.26483137691192e-07 0 0;-0.00114 1.27226702208696e-07 -71133.826080896 -183880.531975666;-0.00108 1.27905175194471e-07 -66956.7018793022 -185442.387824681;-0.00102 1.285182095292e-07 -62745.3213918092 -186909.367921503;-0.00096 1.29065491573191e-07 -58501.839238492 -188280.721732009;-0.0009 1.29546741326837e-07 -54228.4264632307 -189555.747646249;-0.00084 1.29961712573871e-07 -49927.2694229647 -190733.793337405;-0.00078 1.30310193007336e-07 -45600.568669112 -191814.256095535;-0.00072 1.30592004338204e-07 -41250.5378217266 -192796.583135926;-0.00066 1.30807002386589e-07 -36879.4024369692 -193680.271881914;-0.0006 1.30955077155517e-07 -32489.3988684721 -194464.870222007;-0.00054 1.31036152887201e-07 -28082.7731231789 -195149.976741197;-0.00048 1.31050188101799e-07 -23661.7797122458 -195735.240926329;-0.00042 1.30997175618634e-07 -19228.6804975925 -196220.363345432;-0.00036 1.30877142559874e-07 -14785.7435346915 -196605.095800912;-0.0003 1.30690150336648e-07 -10335.2419121891 -196889.241456535;-0.00024 1.30436294617634e-07 -5879.45258895099 -197072.654938135;-0.00018 1.30115705280107e-07 -1420.65522912862 -197155.242407984;-0.00012 1.29728546343498e-07 3038.86896415966 -197136.961612808;-6e-05 1.29275015885471e-07 7496.83841593403 -197017.821905397]  x3=[-0.00192 1.20529575046344e-09 0 0;-0.00186 1.22858992409047e-09 0 0;-0.0018 1.25125552841061e-09 0 0;-0.00174 1.27328096728187e-09 0 0;-0.00168 1.29465497208274e-09 0 0;-0.00162 1.31536660747741e-09 0 0;-0.00156 1.33540527701053e-09 0 0;-0.0015 1.35476072852847e-09 0 0;-0.00144 1.37342305942459e-09 0 0;-0.00138 1.39138272170558e-09 0 0;-0.00132 1.40863052687634e-09 0 0;-0.00126 1.42515765064105e-09 0 0;-0.0012 1.44095563741781e-09 0 0;-0.00114 1.45601640466467e-09 -2523.55538537009 -7088.76443005022;-0.00108 1.47033224701481e-09 -2362.57943032046 -7144.02841745017;-0.00102 1.48389584021876e-09 -2200.39473597884 -7195.63738790528;-0.00096 1.49670024489162e-09 -2037.08427903167 -7243.56493731265;-0.0009 1.50873891006334e-09 -1872.73161212636 -7287.7865450524;-0.00084 1.52000567653039e-09 -1707.42082112418 -7328.27958653289;-0.00078 1.53049478000685e-09 -1541.23648208041 -7365.02334476587;-0.00072 1.54020085407357e-09 -1374.26361797362 -7397.99902096568;-0.00066 1.5491189329237e-09 -1206.58765520641 -7427.18974416706;-0.0006 1.55724445390333e-09 -1038.29437989963 -7452.58057985664;-0.00054 1.56457325984576e-09 -869.469894002605 -7474.15853761371;-0.00048 1.57110160119847e-09 -700.200571241856 -7491.91257775637;-0.00042 1.57682613794139e-09 -530.573012930641 -7505.83361698962;-0.00036 1.58174394129574e-09 -360.674003662149 -7515.91453305255;-0.0003 1.58585249522245e-09 -190.590466908894 -7522.15016836225;-0.00024 1.58914969770943e-09 -20.4094205510611 -7524.53733265246;-0.00018 1.59163386184694e-09 149.782067643448 -7523.07480460581;-0.00012 1.59330371669073e-09 319.896924564497 -7517.7633324787;-6e-05 1.59415840791218e-09 489.848116307923 -7508.60563371839]  x4=[-0.00192 -8.88877600511647e-11 0 0;-0.00186 -6.54866907167683e-11 0 0;-0.0018 -4.20521171813464e-11 0 0;-0.00174 -1.85960290057407e-11 0 0;-0.00168 4.8695732419195e-12 0 0;-0.00162 2.83326841259298e-11 0 0;-0.00156 5.17812994852134e-11 0 0;-0.0015 7.52034225748718e-11 0 0;-0.00144 9.85870702039416e-11 0 0;-0.00138 1.21920278866215e-10 0 0;-0.00132 1.45191110860994e-10 0 0;-0.00126 1.68387660400632e-10 0 0;-0.0012 1.91498059701763e-10 0 0;-0.00114 2.14510485057074e-10 -3803.52800786505 -512.052641091858;-0.00108 2.37413162884531e-10 -3790.97323734558 -597.948379234184;-0.00102 2.60194375750966e-10 -3776.47893486876 -683.538195936878;-0.00096 2.82842468366927e-10 -3760.05251598754 -768.778301868198;-0.0009 3.05345853549744e-10 -3741.70238476137 -853.625086614891;-0.00084 3.27693018151742e-10 -3721.43792945644 -938.035140994095;-0.00078 3.49872528950583e-10 -3699.26951774254 -1021.96527926227;-0.00072 3.71873038498711e-10 -3675.20849138872 -1105.37256120983;-0.00066 3.9368329092892e-10 -3649.26716046065 -1188.21431413013;-0.0006 4.15292127713059e-10 -3621.4587970226 -1270.44815465165;-0.00054 4.36688493370944e-10 -3591.79762834712 -1352.03201042207;-0.00048 4.57861441126545e-10 -3560.29882963619 -1432.92414163327;-0.00042 4.78800138508559e-10 -3526.97851625725 -1513.08316237623;-0.00036 4.99493872892502e-10 -3491.85373549834 -1592.46806181475;-0.0003 5.19932056981488e-10 -3454.9424578463 -1671.03822516741;-0.00024 5.40104234222882e-10 -3416.26356779283 -1748.75345448685;-0.00018 5.60000084158069e-10 -3375.83685417279 -1825.57398922572;-0.00012 5.79609427702589e-10 -3333.68300003986 -1901.46052657898;-6e-05 5.98922232353946e-10 -3289.82357208472 -1976.37424159189]  x5=0.00186628717108595  V1=[7.602e-19 2.561e-08 2.561e-08;377 377 377;2.359 1.029 -0.5418]  V2=[1.596e-23 1.649e-13 1.649e-13;377 377 377;-0.06951 1.06 -0.5113]  I1=[1.208e-21 2.221e-10 2.221e-10;377 377 377;-2.873 2.204 0.633]  I2=[1.433e-21 2.255e-10 2.255e-10;377 377 377;1.006 -0.507 -2.078]  nHarmo=1  Measurements=None  Decoupling=off  VsMag0=0  VrMag0=0  VsAngle0=0  VrAngle0=0  IsMag0=0  IrMag0=0  IsAngle0=0  IrAngle0=0
      settings: LibrarySourceBlock=sps_lib/Power Grid Elements/Distributed Parameters Line
  MPP8 3100 KVA 17KV : spsSynchronousMachinepuStandardLib/Synchronous Machine pu Standard  PresetModel=No  MechanicalLoad=Mechanical power Pm  ShowDetailedParameters=on  RotorType=Salient-pole  Units=per unit standard parameters  MeasurementBus=off  NominalParameters=[3100e6 17000 60]  Reactances1=[ 1.81, 0.3, 0.23, 1.76, 0.65, 0.25, 0.15 ]  Reactances2=[ 1.305, 0.296, 0.252, 0.474, 0.243, 0.18 ]  dAxisTimeConstants=Short-circuit  qAxisTimeConstants=Open-circuit  TimeConstants1="[ 4.4849  0.0681  0.1  ]"  TimeConstants2=[ 8.0, 0.03, 1.0, 0.07 ]  TimeConstants3="[  4.49  0.0681  0.0513  ]"  TimeConstants4=[ 8.0, 0.03, 0.3371, 0.0295 ]  TimeConstants5=[ 1.01, 0.053, 0.1 ]  TimeConstants6=[ 1.3201, 0.023, 1.0, 0.07 ]  TimeConstants7=[0.012 0.003 0.003]  TimeConstants8=[ 1.3201, 0.0231, 0.3371, 0.0295 ]  StatorResistance=2.8544e-3  Mechanical=[3.5 0 32]  PolePairs=20  InitialConditions=[0 -81.9543 0.907703 0.907703 0.907703 -8.76021 -128.76 111.24 1.25655]  SetSaturation=off  Saturation=[0.6404,0.7127,0.8441,0.9214,0.9956,1.082,1.19,1.316,1.457;0.7,0.7698,0.8872,0.9466,0.9969,1.046,1.1,1.151,1.201]  LoadFlowParameters=[1,0,0,0,0]  TsPowergui=0  TsBlock=-1  IterativeModel=Trapezoidal non iterative  IterativeDiscreteModel=Trapezoidal non iterative  BusType=PV  Pref=2900e6  Qref=0  Qmin=-inf  Qmax=inf  PLF=0  QLF=0
  MPP9 4100 MVA 17KV : spsSynchronousMachinepuStandardLib/Synchronous Machine pu Standard  PresetModel=No  MechanicalLoad=Mechanical power Pm  ShowDetailedParameters=on  RotorType=Salient-pole  Units=per unit standard parameters  MeasurementBus=off  NominalParameters="[4100e6  17000   60]"  Reactances1=[ 1.81, 0.3, 0.23, 1.76, 0.65, 0.25, 0.15 ]  Reactances2=[ 1.305, 0.296, 0.252, 0.474, 0.243, 0.18 ]  dAxisTimeConstants=Short-circuit  qAxisTimeConstants=Open-circuit  TimeConstants1="[ 4.4849  0.0681  0.1  ]"  TimeConstants2=[ 8.0, 0.03, 1.0, 0.07 ]  TimeConstants3="[  4.49  0.0681  0.0513  ]"  TimeConstants4=[ 8.0, 0.03, 0.3371, 0.0295 ]  TimeConstants5=[ 1.01, 0.053, 0.1 ]  TimeConstants6=[ 1.3201, 0.023, 1.0, 0.07 ]  TimeConstants7=[0.012 0.003 0.003]  TimeConstants8=[ 1.3201, 0.0231, 0.3371, 0.0295 ]  StatorResistance=2.8544e-3  Mechanical=[3.5 0 32]  PolePairs=20  InitialConditions=[0 -81.9543 0.907703 0.907703 0.907703 -8.76021 -128.76 111.24 1.25655]  SetSaturation=off  Saturation=[0.6404,0.7127,0.8441,0.9214,0.9956,1.082,1.19,1.316,1.457;0.7,0.7698,0.8872,0.9466,0.9969,1.046,1.1,1.151,1.201]  LoadFlowParameters=[1,0,0,0,0]  TsPowergui=0  TsBlock=-1  IterativeModel=Trapezoidal non iterative  IterativeDiscreteModel=Trapezoidal non iterative  BusType=PV  Pref=3500e6  Qref=0  Qmin=-inf  Qmax=inf  PLF=0  QLF=0
  Regulators 7 : Subsystem
  Regulators 8 : Subsystem
  Regulators 9 : Subsystem
  ATL-a : PMIOPort  Side=Right
  ATL-b : PMIOPort  Port=2  Side=Right
  ATL-c : PMIOPort  Port=3  Side=Right
  ORE-a : PMIOPort  Port=4  Side=Left
  ORE-b : PMIOPort  Port=5  Side=Left
  ORE-c : PMIOPort  Port=6  Side=Left
  wires:
  Regulators 8/2(Vf) -> MPP8 3100 KVA 17KV/2
  MPP8 3100 KVA 17KV/1 -> Regulators 8/1(m)
  Regulators 8/1(Pm) -> MPP8 3100 KVA 17KV/1
  Regulators 7/1(Pm) -> MPP7 2700 MVA 17KV/1
  Regulators 7/2(Vf) -> MPP7 2700 MVA 17KV/2
  Regulators 9/1(Pm) -> MPP9 4100 MVA 17KV/1
  Regulators 9/2(Vf) -> MPP9 4100 MVA 17KV/2
  MPP9 4100 MVA 17KV/1 -> Regulators 9/1(m)
  MPP7 2700 MVA 17KV/1 -> Regulators 7/1(m)
  connections:
  ATL-c/RConn1 -- ATL-CAD 447 km/RConn3
  1320 MVar/LConn2 -- MPP7-BMW 330 km/RConn2 -- "2700 MVA 17KV :650KV Transformer "/LConn2
  1320 MVar/LConn1 -- MPP7-BMW 330 km/RConn1 -- Load Flow Bus1/LConn1 -- "2700 MVA 17KV :650KV Transformer "/LConn1
  Cs FER/RConn3 -- FER-LTN 78 km/LConn3 -- 990 Mvar/LConn3
  MPP8 3100 KVA 17KV/RConn2 -- "3100 MVA 17KV :650KV Transformer "/RConn2 -- 155 MW/LConn2
  1320 MVar/LConn3 -- MPP7-BMW 330 km/RConn3 -- "2700 MVA 17KV :650KV Transformer "/LConn3
  Cs FER/LConn3 -- BMW- FER 131 km/RConn3
  "3100 MVA 17KV :650KV Transformer "/RConn3 -- 155 MW/LConn3 -- MPP8 3100 KVA 17KV/RConn3
  Cs FER/RConn2 -- FER-LTN 78 km/LConn2 -- 990 Mvar/LConn2
  ATL-CAD 447 km/RConn1 -- ATL-a/RConn1
  "3100 MVA 17KV :650KV Transformer "/RConn1 -- MPP8 3100 KVA 17KV/RConn1 -- Load Flow Bus2/LConn1 -- 155 MW/LConn1
  Cs FER/RConn1 -- FER-LTN 78 km/LConn1 -- 990 Mvar/LConn1
  Cs FER/LConn2 -- BMW- FER 131 km/RConn2
  Cs FER/LConn1 -- BMW- FER 131 km/RConn1
  ATL-b/RConn1 -- ATL-CAD 447 km/RConn2
  "2700 MVA 17KV :650KV Transformer "/RConn1 -- 135 MW/LConn1 -- MPP7 2700 MVA 17KV/RConn1 -- Load Flow Bus/LConn1
  "2700 MVA 17KV :650KV Transformer "/RConn2 -- 135 MW/LConn2 -- MPP7 2700 MVA 17KV/RConn2
  "2700 MVA 17KV :650KV Transformer "/RConn3 -- 135 MW/LConn3 -- MPP7 2700 MVA 17KV/RConn3
  "4100 MVA 17KV :650KV Transformer "/LConn1 -- LTN 3/RConn1 -- Load Flow Bus6/LConn1
  "4100 MVA 17KV :650KV Transformer "/LConn2 -- LTN 3/RConn2
  "4100 MVA 17KV :650KV Transformer "/LConn3 -- LTN 3/RConn3
  MPP9 4100 MVA 17KV/RConn1 -- Load Flow Bus4/LConn1 -- 205 MW/LConn1 -- "4100 MVA 17KV :650KV Transformer "/RConn1
  MPP9 4100 MVA 17KV/RConn2 -- 205 MW/LConn2 -- "4100 MVA 17KV :650KV Transformer "/RConn2
  MPP9 4100 MVA 17KV/RConn3 -- 205 MW/LConn3 -- "4100 MVA 17KV :650KV Transformer "/RConn3
  BMW- FER 131 km/LConn1 -- BMW- ORE 215 km/LConn1 -- 660 MVar/LConn1 -- CAD 3/RConn1 -- Load Flow Bus3/LConn1 -- "3100 MVA 17KV :650KV Transformer "/LConn1 -- Cs BMW- MPP8/LConn1
  "3100 MVA 17KV :650KV Transformer "/LConn2 -- BMW- ORE 215 km/LConn2 -- 660 MVar/LConn2 -- Cs BMW- MPP8/LConn2 -- BMW- FER 131 km/LConn2 -- CAD 3/RConn2
  BMW- FER 131 km/LConn3 -- 660 MVar/LConn3 -- BMW- ORE 215 km/LConn3 -- Cs BMW- MPP8/LConn3 -- CAD 3/RConn3 -- "3100 MVA 17KV :650KV Transformer "/LConn3
  Cs BMWN/RConn1 -- MPP7-BMW 330 km/LConn1
  Cs BMWN/RConn2 -- MPP7-BMW 330 km/LConn2
  Cs BMWN/RConn3 -- MPP7-BMW 330 km/LConn3
  BMW 1/RConn1 -- Cs BMWN/LConn1
  BMW 1/RConn2 -- Cs BMWN/LConn2
  BMW 1/RConn3 -- Cs BMWN/LConn3
  Cs BMW- MPP8/RConn1 -- BMW 1/LConn1
  Cs BMW- MPP8/RConn2 -- BMW 1/LConn2
  Cs BMW- MPP8/RConn3 -- BMW 1/LConn3
  ATL-CAD 447 km/LConn1 -- 1980 MVar/LConn1 -- CAD 3/LConn1
  ATL-CAD 447 km/LConn2 -- 1980 MVar/LConn2 -- CAD 3/LConn2
  ATL-CAD 447 km/LConn3 -- Load Flow Bus8/LConn1 -- CAD 3/LConn3 -- 1980 MVar/LConn3
  Cs ORED/RConn1 -- ORE-a/RConn1
  Cs ORED/RConn2 -- ORE-b/RConn1
  Cs ORED/RConn3 -- ORE-c/RConn1
  BMW- ORE 215 km/RConn1 -- Load Flow Bus7/LConn1 -- Cs ORED/LConn1
  BMW- ORE 215 km/RConn2 -- Cs ORED/LConn2
  BMW- ORE 215 km/RConn3 -- Cs ORED/LConn3
  Cs LTNN/RConn1 -- FER-LTN 78 km/RConn1
  Cs LTNN/RConn2 -- FER-LTN 78 km/RConn2
  Cs LTNN/RConn3 -- FER-LTN 78 km/RConn3
  LTN 3/LConn1 -- Cs LTNN/LConn1
  LTN 3/LConn2 -- Cs LTNN/LConn2
  LTN 3/LConn3 -- Cs LTNN/LConn3
